simulink model "InertiaWheelSystemTRYTUNING"  (R2013b)
settings: Solver=ode45  StartTime=0.0  StopTime=10.0  RelTol=1e-3
values from neighbouring files (symbols this model uses):
  A = [0 1 0; a/Jw 0 0 ; -(a/Jp) 0 0]    [modelFLAWED.m]
  B = [B_tau B_d]    [modelFLAWED.m]
  C = [1 0 0]    [modelFLAWED.m]
  D = 0    [modelFLAWED.m]
  L = 0.30    (= 0.3)    [modelFLAWED.m]
  lr = 1    [modelFLAWED.m]
undefined symbols (not defined in the file or in its folder): Kt, N, Tdt, Tit, x10, x20, x30, x40
libraries: cstblocks x2, simulink x1
settings Model: Creator=elt11jke  LastModifiedBy=Grivian
settings DataIOCC: SignalLoggingSaveFormat=ModelDataLogs
settings OptimizationCC: ExpressionDepthLimit=2147483647
settings DebuggingCC: MultiTaskDSMMsg=warning  MultiTaskCondExecSysMsg=none  FcnCallInpInsideContextMsg=EnableAllAsWarning  StateNameClashWarn=warning
settings RTWCC: IncludeERTFirstTime=on
settings GRTTargetCC: CodeReplacementLibrary=None  CPPClassGenCompliant=on

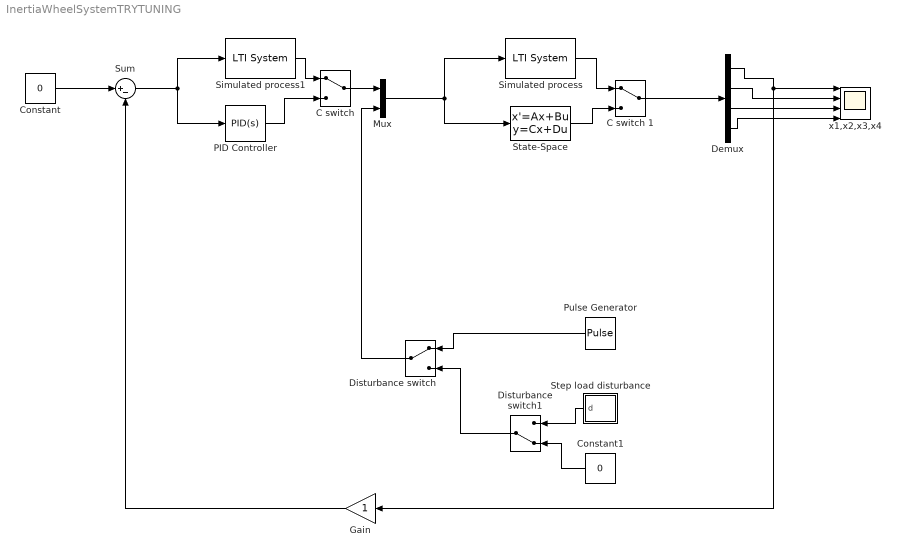
== system InertiaWheelSystemTRYTUNING ==
  "C switch " : ManualSwitch
  C switch 1 : ManualSwitch
  Constant : Constant  Value=0
  Constant1 : Constant  Value=0
  Demux : Demux
  Disturbance switch : ManualSwitch
  Disturbance switch1 : ManualSwitch  CurrentSetting=0
  Gain : Gain
  Mux : Mux  Inputs=2
  PID Controller : simulink/Continuous/PID Controller  Controller=PID  TimeDomain=Continuous-time  SampleTime=1  IntegratorMethod=Forward Euler  FilterMethod=Forward Euler  Form=Parallel  P=Kt  I=Tit  D=Tdt  N=N  InitialConditionSource=internal  InitialConditionForIntegrator=0  InitialConditionForFilter=0  ExternalReset=none  LimitOutput=off  UpperSaturationLimit=inf  LowerSaturationLimit=-inf  LinearizeAsGain=off  AntiWindupMode=none  Kb=1  TrackingMode=off  Kt=1  PParamMin=[]  PParamMax=[]  IParamMin=[]  IParamMax=[]  DParamMin=[]  DParamMax=[]  NParamMin=[]  NParamMax=[]  KbParamMin=[]  KbParamMax=[]  KtParamMin=[]  KtParamMax=[]  POutMin=[]  POutMax=[]  IOutMin=[]  IOutMax=[]  DOutMin=[]  DOutMax=[]  NOutMin=[]  NOutMax=[]  KbOutMin=[]  KbOutMax=[]  KtOutMin=[]  KtOutMax=[]  IntegratorOutMin=[]  IntegratorOutMax=[]  FilterOutMin=[]  FilterOutMax=[]  SumOutMin=[]  SumOutMax=[]  SumI1OutMin=[]  SumI1OutMax=[]  SumI2OutMin=[]  SumI2OutMax=[]  SumI3OutMin=[]  SumI3OutMax=[]  SumDOutMin=[]  SumDOutMax=[]  SaturationOutMin=[]  SaturationOutMax=[]  IntegratorContinuousStateAttributes=''  IntegratorStateMustResolveToSignalObject=off  IntegratorRTWStateStorageClass=Auto  FilterContinuousStateAttributes=''  FilterStateMustResolveToSignalObject=off  FilterRTWStateStorageClass=Auto
  Pulse Generator : DiscretePulseGenerator  PulseType=Time based  Amplitude=0.01  Period=3  PulseWidth=5
  Simulated process : cstblocks/LTI System  sys=PinSF  IC=[]
  Simulated process1 : cstblocks/LTI System  sys=Cin  IC=[]
  State-Space : StateSpace  A=A-B*L  B=B*lr  C=C  D=D  X0=[x10 x20 x30 x40]  ContinuousStateAttributes={'Pendulum', 'Motor'}
  Step load disturbance : Subsystem
  Sum : Sum  Inputs=|+-
  "x1,x2,x3,x4 " : Scope  NumInputPorts=4
      settings: ShowLegends=on  YMin=-5~-5~-5~-5  YMax=5~5~5~5
  wires:
  Gain/1 -> Sum/2
  Constant/1 -> Sum/1
  Demux/1 -> Gain/1, "x1,x2,x3,x4 "/1
  Demux/2 -> "x1,x2,x3,x4 "/2
  Demux/3 -> "x1,x2,x3,x4 "/3
  Demux/4 -> "x1,x2,x3,x4 "/4
  Pulse Generator/1 -> Disturbance switch/1
  Disturbance switch/1 -> Mux/2
  Sum/1 -> Simulated process1/1, PID Controller/1
  Simulated process1/1 -> "C switch "/1
  PID Controller/1 -> "C switch "/2
  "C switch "/1 -> Mux/1
  Mux/1 -> State-Space/1, Simulated process/1
  C switch 1/1 -> Demux/1
  Step load disturbance/1(d) -> Disturbance switch1/1
  Constant1/1 -> Disturbance switch1/2
  Disturbance switch1/1 -> Disturbance switch/2
  Simulated process/1 -> C switch 1/1
  State-Space/1 -> C switch 1/2

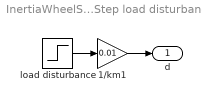
== system InertiaWheelSystemTRYTUNING/Step load disturbance ==
  1/km1 : Gain  Gain=0.01  SaturateOnIntegerOverflow=on  OutDataTypeStr=Inherit: Same as input  ParamDataTypeStr=Inherit: Same as input
  load disturbance : Step  Time=5  After=-0.15  SampleTime=0
  d : Outport
  wires:
  load disturbance/1 -> 1/km1/1
  1/km1/1 -> d/1
